simulink model "ex04_model_ADC_R2023a"  (R2023a)
settings: Solver=VariableStepAuto  StartTime=0.0  StopTime=0.01  FixedStep=Ts  MaxStep=1e-4  MinStep=1e-5  RelTol=1e-3
values from neighbouring files (symbols this model uses):
  omega_0 = 2*pi*Fc_0    (= 3141.59265359)    [ex04_config_ADC.m]
  phi_0 = pi/4    (= 0.785398163397)    [ex02.m]    (also in ex04_config_ADC.m = 0)
  Ts = 1/Fs    (= 6.25e-05)    [ex00.m]    (also in ex01.m = 0.00025; ex02.m = 0.00025; ex04_config_ADC.m = 0.00025)
libraries: dspsigops x1, dspquant2 x1
settings Model: Creator=daniele  LastModifiedBy=mluser
settings SolverCC: InitialStep=1e-5  AlgebraicLoopSolver=TrustRegion
settings DataIOCC: ReturnWorkspaceOutputs=off
settings OptimizationCC: ReuseModelBlockBuffer=off
settings DebuggingCC: UnconnectedInputMsg=warning  UnconnectedOutputMsg=warning  UnconnectedLineMsg=warning  ArithmeticOperatorsInVariantConditions=warning
settings ModelReferenceCC: EnableRefExpFcnMdlSchedulingChecks=on
settings SFSimCC: CustomCodeUndefinedFunction=UseInterfaceOnly
settings RTWCC: DLArmComputeVersion=19.05

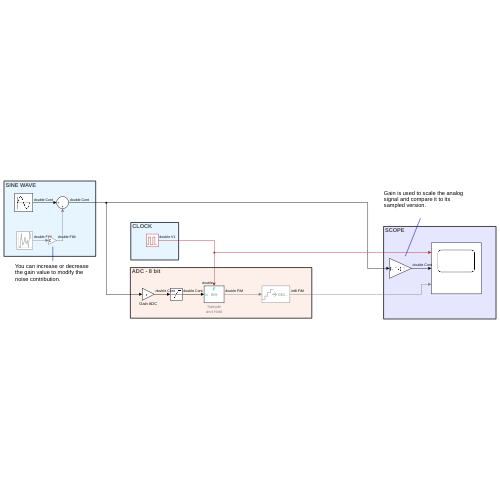
[thumbnail: Simulink's stored preview of the top-level diagram]
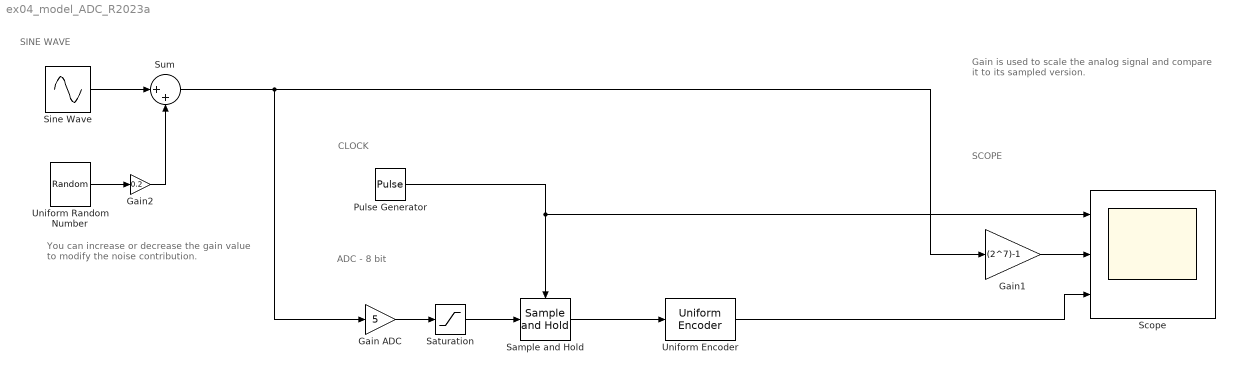
== system ex04_model_ADC_R2023a ==
  note: You can increase or decrease the gain value to modify the noise contribution.
  note: Gain is used to scale the analog signal and compare it to its sampled version.
  note: SCOPE
  note: CLOCK
  note: ADC - 8 bit
  note: SINE WAVE
  Gain ADC : Gain  Gain=5
  Gain1 : Gain  Gain=(2^7)-1
  Gain2 : Gain  Gain=0.2
  Pulse Generator : DiscretePulseGenerator  PulseType=Time based  Period=Ts  PulseWidth=50
  Sample and Hold : dspsigops/Sample and Hold  trig=Rising edge  initCond=0  latchinput=off
  Saturation : Saturate  UpperLimit=5  LowerLimit=-5  ZeroCross=off
  Scope : Scope  NumInputPorts=3
  Sine Wave : Sin  Frequency=omega_0  Phase=phi_0  SampleTime=0
  Sum : Sum  Inputs=|++
  Uniform Encoder : dspquant2/Uniform Encoder  peak=5  bits=8  otype=Signed integer
  Uniform Random Number : UniformRandomNumber  SampleTime=0
  wires:
  Saturation/1 -> Sample and Hold/1
  Sum/1 -> Gain ADC/1, Gain1/1
  Sample and Hold/1 -> Uniform Encoder/1
  Pulse Generator/1 -> Sample and Hold/Trigger, Scope/1
  Uniform Encoder/1 -> Scope/3
  Gain1/1 -> Scope/2
  Gain ADC/1 -> Saturation/1
  Sine Wave/1 -> Sum/1
  Uniform Random Number/1 -> Gain2/1
  Gain2/1 -> Sum/2
